simulink model "UAV_Dynamics"  (R2024b)
settings: Solver=ode4  StartTime=0.0  StopTime=10.0  RelTol=1e-3
undefined symbols (not defined in the file): contact, control, ddx, ddy, ddz, dragCoeffMov, dx, dy, dz, fractalcoef, g, m_to_mm, mass, p, pitch, q, r, ref_height, ref_lat, ref_lon, roll, rotorDir, rotorPositions, rotorThrustMax, rotorTimeConst, rotorTorqueMax, SampleTime, windVel, X, Y, yaw, Z
libraries: aerolibatmos2 x1, sensorgpslib x1, robotcorelib x1, mspsensorlib x1, shared6dof x1, simulink x1
settings Model: Creator=The MathWorks, Inc.  LastModifiedBy=davi1
settings SolverCC: ZeroCrossControl=EnableAll  MaxZcPerStep=1
settings OptimizationCC: ReuseModelBlockBuffer=off
settings ModelReferenceCC: EnableRefExpFcnMdlSchedulingChecks=on
settings RTWCC: GPUComputeCapability=3.5  DLArmComputeVersion=19.05

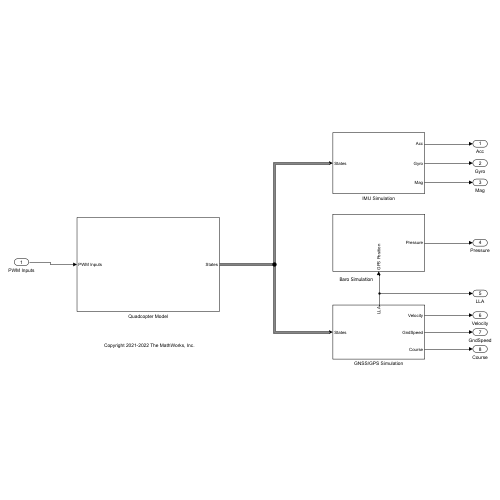
[thumbnail: Simulink's stored preview of the top-level diagram]
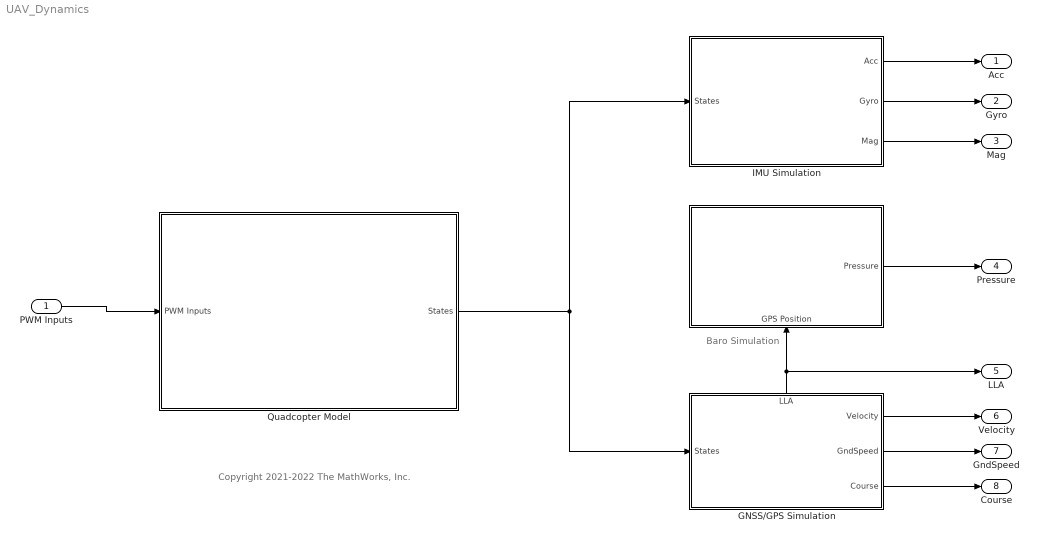
== system UAV_Dynamics ==
  note: Baro Simulation
  note: Copyright 2021-2022 The MathWorks, Inc.
  PWM Inputs : Inport
  " " : Subsystem
      settings: PortSchema="{\"entries\":[{\"content\":{\"sides\":[{\"content\":{\"connectorIds\":[]},\"type\":\"ConnectorPlacement.EquallySpacedRectSide\",\"uuid\":\"7ecc8b21-8f8f-4144-826a-6b68e30dbf7d\"},{\"content\":{\"connectorIds\":[\"Out1\"],\"side\":\"RIGHT\"},\"type\":\"ConnectorPlacement.EquallySpacedRectSide\",\"uuid\":\"81a1dd55-8330-4386-9921-36c0eb60d526\"},{\"content\":{\"connectorIds\":[],\"side\":\"TOP\"},\"type\":\"ConnectorPlacement.EquallySpacedRectSide\",\"uuid\":\"b99caff5-b40d-407d-b30e-35210c1aee1d\"},{\"content\":{\"connectorIds\":[\"In1\"],\"side\":\"BOTTOM\"},\"type\":\"ConnectorPlacement.EquallySpacedRectSide\",\"uuid\":\"18bfda3d-4fab-4e61-9ebc-e384e51de306\"}]},\"type\":\"ConnectorPlacement.EquallySpacedConnector\",\"uuid\":\"17ab4e96-b761-4c62-a0bb-ab626dac3eaa\"}],\"packageUris\":[\"http://schema.mathworks.com/mf0/Connector/R2020b\"],\"version\":\"1.0\"}"
  GNSS/GPS Simulation : Subsystem
      settings: PortSchema="{\"entries\":[{\"content\":{\"sides\":[{\"content\":{\"connectorIds\":[\"In1\"]},\"type\":\"ConnectorPlacement.EquallySpacedRectSide\",\"uuid\":\"4934e8ff-5d4b-4e11-968d-c23bd62383a0\"},{\"content\":{\"connectorIds\":[\"Out1\",\"Out2\",\"Out3\"],\"side\":\"RIGHT\"},\"type\":\"ConnectorPlacement.EquallySpacedRectSide\",\"uuid\":\"9ec8bc0a-2d3c-4dca-835c-010ac29b6ebc\"},{\"content\":{\"connectorIds\":[\"Out4\"],\"side\":\"TOP\"},\"type\":\"ConnectorPlacement.EquallySpacedRectSide\",\"uuid\":\"04f09eb4-1bd9-450e-b951-47054bdd92ad\"}]},\"type\":\"ConnectorPlacement.EquallySpacedConnector\",\"uuid\":\"9a5920cf-a58d-4c98-839b-fbac94edbe7e\"}],\"packageUris\":[\"http://schema.mathworks.com/mf0/Connector/R2020b\"],\"version\":\"1.0\"}"
  IMU Simulation : Subsystem
  Quadcopter Model : Subsystem
  Acc : Outport
  Gyro : Outport  Port=2
  Mag : Outport  Port=3
  Pressure : Outport  Port=4
  LLA : Outport  Port=5
  Velocity : Outport  Port=6
  GndSpeed : Outport  Port=7
  Course : Outport  Port=8
  wires:
  Quadcopter Model/1(States) -> IMU Simulation/1(States), GNSS/GPS Simulation/1(States)
  PWM Inputs/1 -> Quadcopter Model/1(PWM Inputs)
  IMU Simulation/1(Acc) -> Acc/1
  IMU Simulation/2(Gyro) -> Gyro/1
  IMU Simulation/3(Mag) -> Mag/1
  " "/1(Pressure) -> Pressure/1
  GNSS/GPS Simulation/1(Velocity) -> Velocity/1
  GNSS/GPS Simulation/2(GndSpeed) -> GndSpeed/1
  GNSS/GPS Simulation/3(Course) -> Course/1
  GNSS/GPS Simulation/4(LLA) -> LLA/1, " "/1(GPS Position)

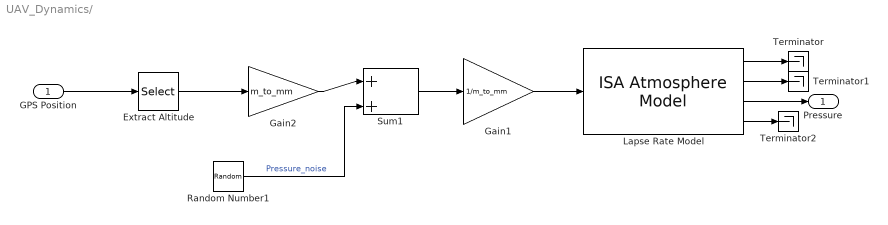
== system UAV_Dynamics/  ==
  GPS Position : Inport
  Extract Altitude : Selector  InputPortWidth=3  IndexOptions=Index vector (dialog)  Indices=[3]  OutputSizes=1
  Gain1 : Gain  Gain=1/m_to_mm
  Gain2 : Gain  Gain=m_to_mm
  Lapse Rate Model : aerolibatmos2/ISA Atmosphere Model  useExtended=off  action=Warning  custom=on  viscosityOut=off  g=9.80665  gamma=1.4  R=287.0531  L=0.0065  h_trop=11000  h_strat=20000  rho0=1.225  P0=101325  T0=288.15  h0=0  S=110.4  Tref=273.15  muref=1.716e-5
  Random Number1 : RandomNumber  Variance=10000  Seed=10  SampleTime=SampleTime
  Sum1 : Sum  Inputs=|++
  Terminator : Terminator
  Terminator1 : Terminator
  Terminator2 : Terminator
  Pressure : Outport
  wires:
  Lapse Rate Model/2 -> Terminator1/1
  Lapse Rate Model/4 -> Terminator2/1
  Lapse Rate Model/1 -> Terminator/1
  Lapse Rate Model/3 -> Pressure/1
  Sum1/1 -> Gain1/1
  Gain2/1 -> Sum1/1
  Extract Altitude/1 -> Gain2/1
  Gain1/1 -> Lapse Rate Model/1
  GPS Position/1 -> Extract Altitude/1
  Random Number1/1 -> Sum1/2  "Pressure_noise"

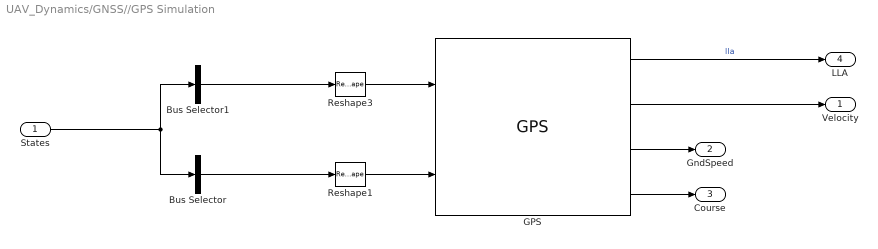
== system UAV_Dynamics/GNSS//GPS Simulation ==
  States : Inport
  Bus Selector : BusSelector  OutputSignals=dx,dy,dz  OutputAsBus=on
  Bus Selector1 : BusSelector  OutputSignals=X,Y,Z  OutputAsBus=on
  GPS : sensorgpslib/GPS  DispRefFrame=NED  PositionInputFormat=Local  ReferenceLocation=[ref_lat ref_lon ref_height]  HorizontalPositionAccuracy=0.01  VerticalPositionAccuracy=0.01  VelocityAccuracy=0.01  DecayFactor=0.99  SeedDouble=67  SimulateUsing=Interpreted execution
  Reshape1 : Reshape  OutputDimensionality=Row vector (2-D)
  Reshape3 : Reshape  OutputDimensionality=Row vector (2-D)
  Velocity : Outport
  GndSpeed : Outport  Port=2
  Course : Outport  Port=3
  LLA : Outport  Port=4
  wires:
  Reshape3/1 -> GPS/1
  GPS/1 -> LLA/1  "lla"
  Bus Selector1/1 -> Reshape3/1
  Bus Selector/1 -> Reshape1/1
  Reshape1/1 -> GPS/2
  GPS/2 -> Velocity/1
  States/1 -> Bus Selector/1, Bus Selector1/1
  GPS/3 -> GndSpeed/1
  GPS/4 -> Course/1

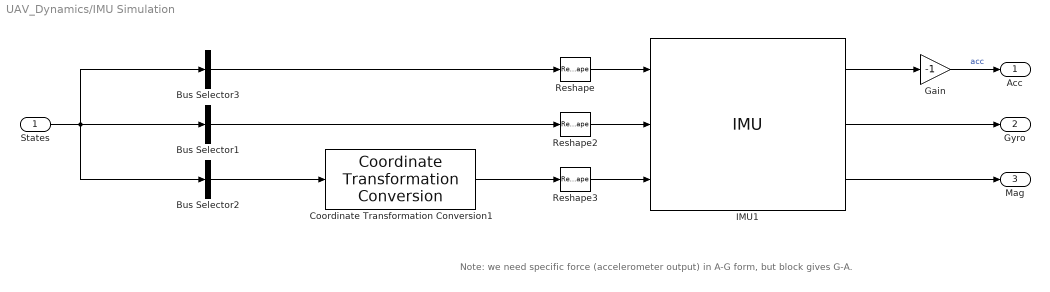
== system UAV_Dynamics/IMU Simulation ==
  note: Note:
      | we need specific force (accelerometer output) in A-G form, but block gives G-A.
  States : Inport
  Bus Selector1 : BusSelector  OutputSignals=p,q,r  OutputAsBus=on
  Bus Selector2 : BusSelector  OutputSignals=yaw,pitch,roll  OutputAsBus=on
  Bus Selector3 : BusSelector  OutputSignals=ddx,ddy,ddz  OutputAsBus=on
  Coordinate Transformation Conversion1 : robotcorelib/Coordinate Transformation Conversion  InputRepresentation=Euler Angles  InputEulerSequence=ZYX  ShowTrVecInputPort=on  OutputRepresentation=Quaternion  OutputEulerSequence=ZYX  ShowTrVecOutputPort=on  SimulateUsing=Interpreted execution
  Gain : Gain  Gain=-1
  IMU1 : mspsensorlib/IMU  DispRefFrame=NED  TemperaturePort=off  Temperature=25  MagneticFieldPort=off  MagneticFieldNED=[21.5 1.16 43.1]  MagneticFieldENU=[ -2.4169, 27.5550, 16.0849 ]  SeedDouble=87254  SimulateUsing=Interpreted execution  AccelParamsMeasurementRange=Inf  AccelParamsResolution=0  AccelParamsConstantBias=[ 0, 0, 0 ]  AccelParamsAxesMisalignment=[ 0, 0, 0 ]  AccelParamsNoiseDensity=0.0003  AccelParamsBiasInstability=[ 0, 0, 0 ]  AccelParamsBiasInstabilityNumerator=fractalcoef().Numerator  AccelParamsBiasInstabilityDenominator=fractalcoef().Denominator  AccelParamsRandomWalk=[ 0, 0, 0 ]  AccelParamsNoiseType=double-sided  AccelParamsTemperatureBias=[ 0, 0, 0 ]  AccelParamsTemperatureScaleFactor=[ 0, 0, 0 ]  GyroParamsMeasurementRange=Inf  GyroParamsResolution=0  GyroParamsConstantBias=[ 0, 0, 0 ]  GyroParamsAxesMisalignment=[ 0, 0, 0 ]  GyroParamsAccelerationBias=0.0001  GyroParamsNoiseDensity=0.01  GyroParamsBiasInstability=[ 0, 0, 0 ]  GyroParamsBiasInstabilityNumerator=fractalcoef().Numerator  GyroParamsBiasInstabilityDenominator=fractalcoef().Denominator  GyroParamsRandomWalk=[ 0, 0, 0 ]  GyroParamsNoiseType=double-sided  GyroParamsTemperatureBias=[ 0, 0, 0 ]  GyroParamsTemperatureScaleFactor=[ 0, 0, 0 ]  MagParamsMeasurementRange=Inf  MagParamsResolution=0  MagParamsConstantBias=[ 0, 0, 0 ]  MagParamsAxesMisalignment=[ 0, 0, 0 ]  MagParamsNoiseDensity=0.0005  MagParamsBiasInstability=[ 0, 0, 0 ]  MagParamsBiasInstabilityNumerator=fractalcoef().Numerator  MagParamsBiasInstabilityDenominator=fractalcoef().Denominator  MagParamsRandomWalk=[ 0, 0, 0 ]  MagParamsNoiseType=double-sided  MagParamsTemperatureBias=[ 0, 0, 0 ]  MagParamsTemperatureScaleFactor=[ 0, 0, 0 ]
  Reshape : Reshape  OutputDimensionality=Row vector (2-D)
  Reshape2 : Reshape  OutputDimensionality=Row vector (2-D)
  Reshape3 : Reshape  OutputDimensionality=Row vector (2-D)
  Acc : Outport
  Gyro : Outport  Port=2
  Mag : Outport  Port=3
  wires:
  Coordinate Transformation Conversion1/1 -> Reshape3/1
  Reshape3/1 -> IMU1/3
  IMU1/3 -> Mag/1
  IMU1/2 -> Gyro/1
  Reshape/1 -> IMU1/1
  Bus Selector3/1 -> Reshape/1
  IMU1/1 -> Gain/1
  Bus Selector1/1 -> Reshape2/1
  Bus Selector2/1 -> Coordinate Transformation Conversion1/1
  Reshape2/1 -> IMU1/2
  States/1 -> Bus Selector1/1, Bus Selector2/1, Bus Selector3/1
  Gain/1 -> Acc/1  "acc"

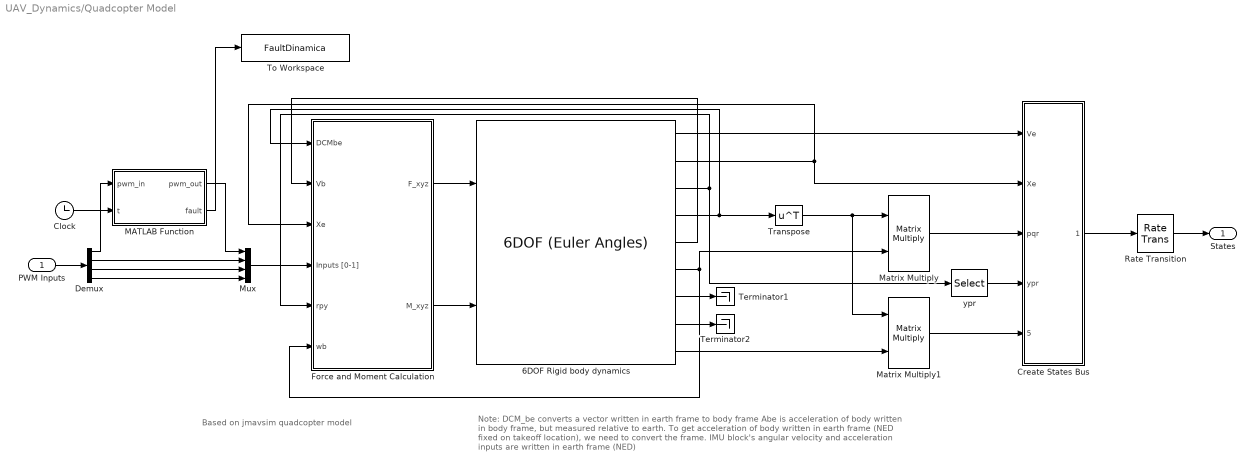
== system UAV_Dynamics/Quadcopter Model ==
  note: Note:
      | DCM_be converts a vector written in earth frame to body frame
      | Abe is acceleration of body written in body frame, but measured relative to earth.
      | To get acceleration of body written in earth frame (NED fixed on takeoff location), we need to convert the frame.
      | IMU block's angular velocity and acceleration inputs are written in earth frame (NED)
  note: Based on jmavsim quadcopter model
  PWM Inputs : Inport
  "6DOF Rigid body dynamics " : shared6dof/6DOF (Euler Angles)  units=Metric (MKS)  mtype=Fixed  rep=Quaternion  xme_0=init.posNED  Vm_0=init.vb  eul_0=init.euler  pm_0=init.angRates  mass_0=mass  mass_e=0.5  mass_f=2.0  inertia=inertia  inertia_e=eye(3)  inertia_f=2*eye(3)  k_quat=1  vre_flag=on  abi_flag=on  aMode=aMode  xme_statename=''  Vm_statename=''  eul_statename=''  quat_statename=''  pm_statename=''  mass_statename=''
  Clock : Clock
  Create States Bus : Subsystem
  Demux : Demux
  Force and Moment Calculation : Subsystem
  MATLAB Function : MATLAB Function  TreatAsAtomicUnit=on
  Matrix Multiply : Product  Multiplication=Matrix(*)
  Matrix Multiply1 : Product  Multiplication=Matrix(*)
  Mux : Mux
  Rate Transition : RateTransition  OutPortSampleTime=SampleTime
  Terminator1 : Terminator
  Terminator2 : Terminator
  To Workspace : ToWorkspace  VariableName=FaultDinamica  SaveFormat=Structure With Time  SampleTime=-1
  Transpose : Math  Operator=transpose
  ypr : Selector  InputPortWidth=3  IndexOptions=Index vector (dialog)  Indices=[3 2 1]  OutputSizes=1
  States : Outport
  wires:
  Matrix Multiply/1 -> Create States Bus/3(pqr)
  "6DOF Rigid body dynamics "/6 -> Matrix Multiply/2, Force and Moment Calculation/6(wb)
  Force and Moment Calculation/1(F_xyz) -> "6DOF Rigid body dynamics "/1
  "6DOF Rigid body dynamics "/9 -> Matrix Multiply1/2
  Transpose/1 -> Matrix Multiply1/1, Matrix Multiply/1
  "6DOF Rigid body dynamics "/5 -> Force and Moment Calculation/2(Vb)
  ypr/1 -> Create States Bus/4(ypr)
  "6DOF Rigid body dynamics "/2 -> Force and Moment Calculation/3(Xe), Create States Bus/2(Xe)
  "6DOF Rigid body dynamics "/3 -> Force and Moment Calculation/5(rpy), ypr/1
  Rate Transition/1 -> States/1
  Create States Bus/1(States) -> Rate Transition/1
  "6DOF Rigid body dynamics "/7 -> Terminator1/1
  "6DOF Rigid body dynamics "/1 -> Create States Bus/1(Ve)
  "6DOF Rigid body dynamics "/8 -> Terminator2/1
  Force and Moment Calculation/2(M_xyz) -> "6DOF Rigid body dynamics "/2
  "6DOF Rigid body dynamics "/4 -> Force and Moment Calculation/1(DCMbe), Transpose/1
  Matrix Multiply1/1 -> Create States Bus/5(acc_lnav)
  PWM Inputs/1 -> Demux/1
  Mux/1 -> Force and Moment Calculation/4(Inputs [0-1])
  Demux/4 -> Mux/4
  Demux/3 -> Mux/3
  Demux/2 -> Mux/2
  MATLAB Function/1(pwm_out) -> Mux/1
  Demux/1 -> MATLAB Function/1(pwm_in)
  Clock/1 -> MATLAB Function/2(t)
  MATLAB Function/2(fault) -> To Workspace/1

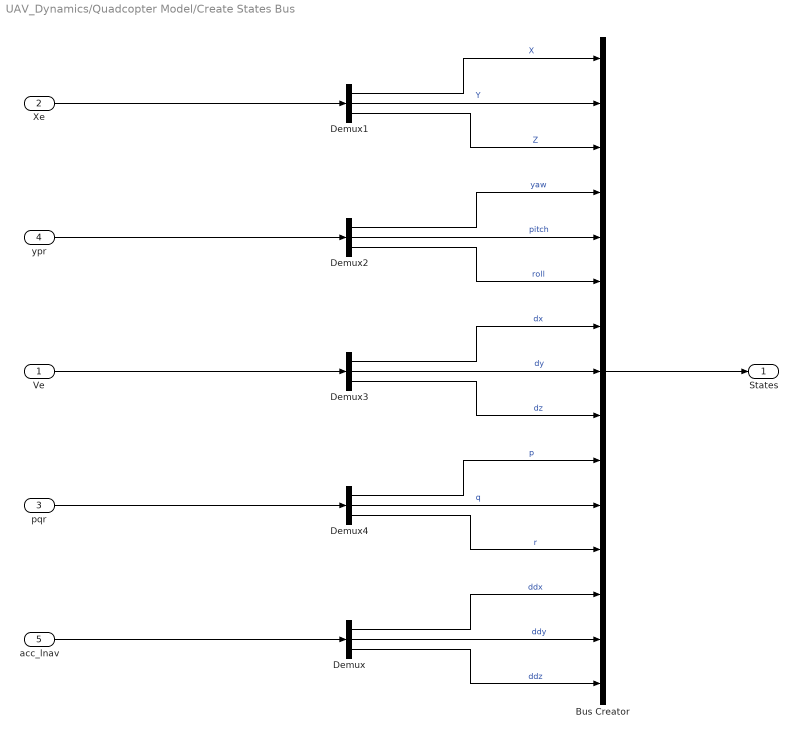
== system UAV_Dynamics/Quadcopter Model/Create States Bus ==
  Ve : Inport
  Xe : Inport  Port=2
  pqr : Inport  Port=3
  ypr : Inport  Port=4
  acc_lnav : Inport  Port=5
  Bus Creator : BusCreator  Inputs=X,Y,Z,yaw,pitch,roll,dx,dy,dz,p,q,r,ddx,ddy,ddz
  Demux{,1..4} (5 alike) : Demux  Outputs=3
  States : Outport
  wires:
  Demux1/1 -> Bus Creator/1  "X"
  Demux1/2 -> Bus Creator/2  "Y"
  ypr/1 -> Demux2/1
  Demux2/2 -> Bus Creator/5  "pitch"
  Demux3/2 -> Bus Creator/8  "dy"
  Demux2/3 -> Bus Creator/6  "roll"
  pqr/1 -> Demux4/1
  Ve/1 -> Demux3/1
  Demux2/1 -> Bus Creator/4  "yaw"
  Demux1/3 -> Bus Creator/3  "Z"
  Demux3/1 -> Bus Creator/7  "dx"
  Demux4/2 -> Bus Creator/11  "q"
  Demux3/3 -> Bus Creator/9  "dz"
  Demux4/3 -> Bus Creator/12  "r"
  Demux4/1 -> Bus Creator/10  "p"
  Bus Creator/1 -> States/1
  Xe/1 -> Demux1/1
  acc_lnav/1 -> Demux/1
  Demux/3 -> Bus Creator/15  "ddz"
  Demux/2 -> Bus Creator/14  "ddy"
  Demux/1 -> Bus Creator/13  "ddx"

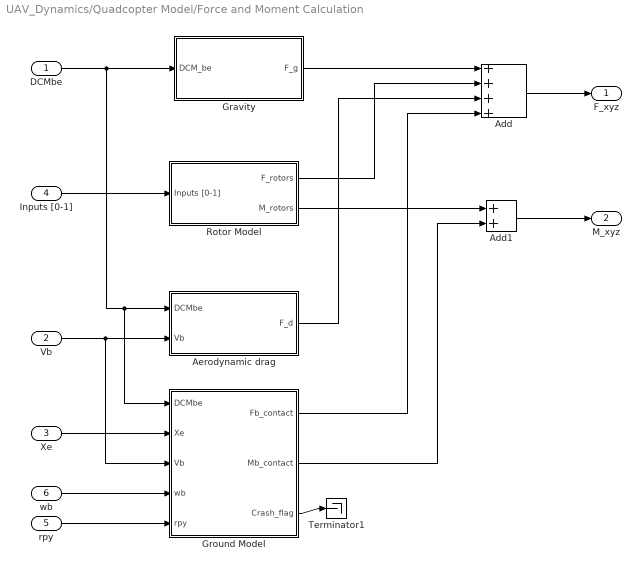
== system UAV_Dynamics/Quadcopter Model/Force and Moment Calculation ==
  DCMbe : Inport
  Vb : Inport  Port=2
  Xe : Inport  Port=3
  Inputs [0-1] : Inport  Port=4
  rpy : Inport  Port=5
  wb : Inport  Port=6
  Add : Sum  Inputs=++++
  Add1 : Sum
  Aerodynamic drag : Subsystem
  Gravity : Subsystem
  Ground Model : Subsystem
  Rotor Model : Subsystem
  Terminator1 : Terminator
  F_xyz : Outport
  M_xyz : Outport  Port=2
  wires:
  Inputs [0-1]/1 -> Rotor Model/1(Inputs [0-1])
  DCMbe/1 -> Ground Model/1(DCMbe), Aerodynamic drag/1(DCMbe), Gravity/1(DCM_be)
  Gravity/1(F_g) -> Add/1
  Add/1 -> F_xyz/1
  Vb/1 -> Ground Model/3(Vb), Aerodynamic drag/2(Vb)
  Rotor Model/1(F_rotors) -> Add/2
  Aerodynamic drag/1(F_d) -> Add/3
  Xe/1 -> Ground Model/2(Xe)
  wb/1 -> Ground Model/4(wb)
  rpy/1 -> Ground Model/5(rpy)
  Rotor Model/2(M_rotors) -> Add1/1
  Ground Model/2(Mb_contact) -> Add1/2
  Add1/1 -> M_xyz/1
  Ground Model/1(Fb_contact) -> Add/4
  Ground Model/3(Crash_flag) -> Terminator1/1

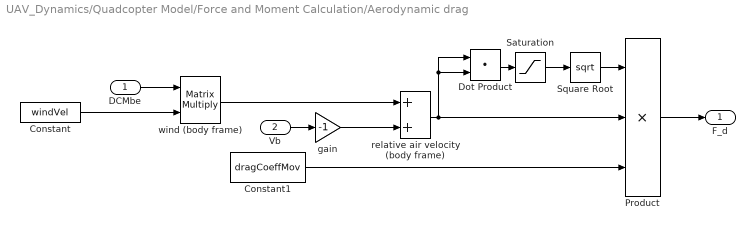
== system UAV_Dynamics/Quadcopter Model/Force and Moment Calculation/Aerodynamic drag ==
  DCMbe : Inport
  Vb : Inport  Port=2
  Constant : Constant  Value=windVel
  Constant1 : Constant  Value=dragCoeffMov
  Dot Product : DotProduct  OutDataTypeStr=Inherit: Inherit via internal rule
  Product : Product  Inputs=3
  Saturation : Saturate  UpperLimit=inf  LowerLimit=0.0001
  Square Root : Sqrt
  gain : Gain  Gain=-1
  relative air velocity (body frame) : Sum
  wind (body frame) : Product  Multiplication=Matrix(*)
  F_d : Outport
  wires:
  relative air velocity (body frame)/1 -> Dot Product/2, Dot Product/1, Product/2
  DCMbe/1 -> wind (body frame)/1
  Product/1 -> F_d/1
  Saturation/1 -> Square Root/1
  Vb/1 -> gain/1
  Dot Product/1 -> Saturation/1
  Square Root/1 -> Product/1
  wind (body frame)/1 -> relative air velocity (body frame)/1
  gain/1 -> relative air velocity (body frame)/2
  Constant1/1 -> Product/3
  Constant/1 -> wind (body frame)/2

== system UAV_Dynamics/Quadcopter Model/Force and Moment Calculation/Gravity ==
  DCM_be : Inport
  Constant : Constant  Value=[0 0 g]'
  Gain : Gain  Gain=mass
  Matrix Multiply : Product  Multiplication=Matrix(*)
  F_g : Outport
  wires:
  Matrix Multiply/1 -> Gain/1
  Constant/1 -> Matrix Multiply/2
  DCM_be/1 -> Matrix Multiply/1
  Gain/1 -> F_g/1

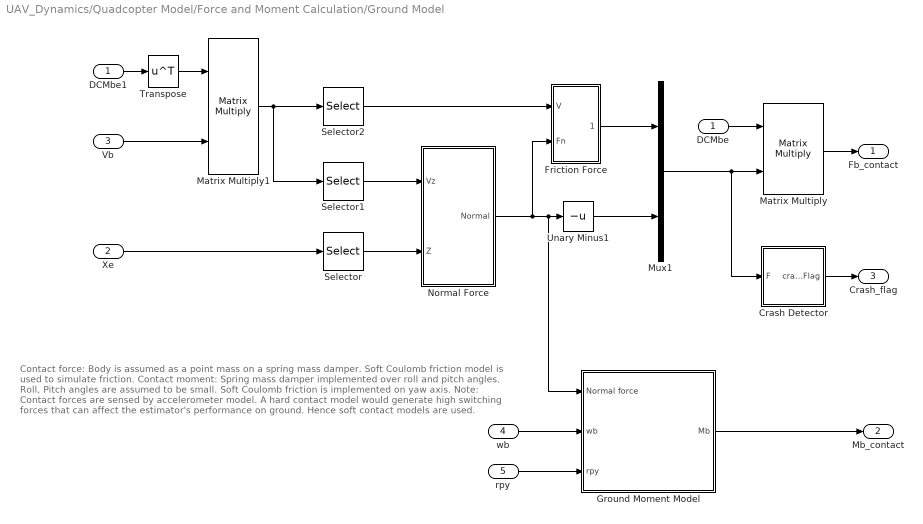
== system UAV_Dynamics/Quadcopter Model/Force and Moment Calculation/Ground Model ==
  note: Contact force:
      | Body is assumed as a point mass on a spring mass damper. Soft Coulomb friction model is used to simulate friction.
      |
      | Contact moment:
      | Spring mass damper implemented over roll and pitch angles. Roll, Pitch angles are assumed to be small.
      | Soft Coulomb friction is implemented on yaw axis.
      |
      | Note:
      | Contact forces are sensed by accelerometer model. A hard contact model would generate high switching forces that can affect the estimator's performance on ground. Hence soft contact models are used.
  DCMbe : Inport
  Xe : Inport  Port=2
  Vb : Inport  Port=3
  wb : Inport  Port=4
  rpy : Inport  Port=5
  Crash Detector : Subsystem
  DCMbe1 : InportShadow
  Friction Force : Subsystem
  Ground Moment Model : Subsystem
  Matrix Multiply : Product  Multiplication=Matrix(*)
  Matrix Multiply1 : Product  Multiplication=Matrix(*)
  Mux1 : Mux  Inputs=2
  Normal Force : Subsystem
  Selector : Selector  InputPortWidth=3  IndexOptions=Index vector (dialog)  Indices=[3]  OutputSizes=1
  Selector1 : Selector  InputPortWidth=3  IndexOptions=Index vector (dialog)  Indices=[3]  OutputSizes=1
  Selector2 : Selector  InputPortWidth=3  IndexOptions=Index vector (dialog)  Indices=[1,2]  OutputSizes=1
  Transpose : Math  Operator=transpose
  Unary Minus1 : UnaryMinus
  Fb_contact : Outport
  Mb_contact : Outport  Port=2
  Crash_flag : Outport  Port=3
  wires:
  Crash Detector/1(crashFlag) -> Crash_flag/1
  Xe/1 -> Selector/1
  Selector1/1 -> Normal Force/1(Vz)
  Selector/1 -> Normal Force/2(Z)
  DCMbe/1 -> Matrix Multiply/1
  Matrix Multiply/1 -> Fb_contact/1
  Normal Force/1(Normal) -> Ground Moment Model/1(Normal force), Unary Minus1/1, Friction Force/2(Fn)
  Mux1/1 -> Crash Detector/1(F), Matrix Multiply/2
  Unary Minus1/1 -> Mux1/2
  Selector2/1 -> Friction Force/1(V)
  Friction Force/1(Friction) -> Mux1/1
  DCMbe1/1 -> Transpose/1
  Transpose/1 -> Matrix Multiply1/1
  Vb/1 -> Matrix Multiply1/2
  Matrix Multiply1/1 -> Selector1/1, Selector2/1
  wb/1 -> Ground Moment Model/2(wb)
  rpy/1 -> Ground Moment Model/3(rpy)
  Ground Moment Model/1(Mb) -> Mb_contact/1

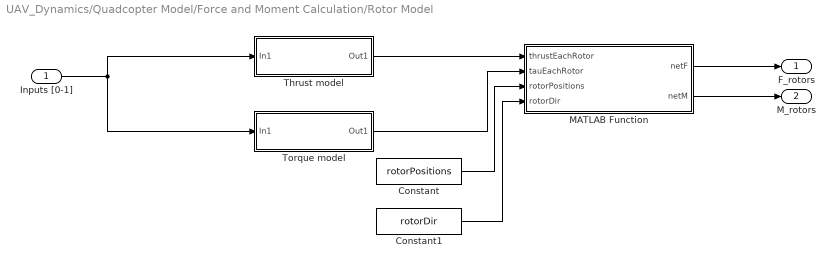
== system UAV_Dynamics/Quadcopter Model/Force and Moment Calculation/Rotor Model ==
  Inputs [0-1] : Inport
  Constant : Constant  Value=rotorPositions
  Constant1 : Constant  Value=rotorDir
  MATLAB Function : MATLAB Function  TreatAsAtomicUnit=on
  Thrust model : Subsystem
  Torque model : Subsystem
  F_rotors : Outport
  M_rotors : Outport  Port=2
  wires:
  Inputs [0-1]/1 -> Torque model/1(In1), Thrust model/1(In1)
  MATLAB Function/1(netF) -> F_rotors/1
  MATLAB Function/2(netM) -> M_rotors/1
  Constant/1 -> MATLAB Function/3(rotorPositions)
  Constant1/1 -> MATLAB Function/4(rotorDir)
  Torque model/1(Out1) -> MATLAB Function/2(tauEachRotor)
  Thrust model/1(Out1) -> MATLAB Function/1(thrustEachRotor)

== system UAV_Dynamics/Quadcopter Model/Force and Moment Calculation/Ground Model/Crash Detector ==
  F : Inport
  Compare To Constant : simulink/Logic and Bit Operations/Compare To Constant  relop=>  const=100  OutDataTypeStr=boolean
  Gain : Gain  Gain=1/mass/g
  norm1 : Subsystem
  crashFlag : Outport
  wires:
  F/1 -> norm1/1(F)
  norm1/1(Out1) -> Gain/1
  Compare To Constant/1 -> crashFlag/1
  Gain/1 -> Compare To Constant/1  "g's"

== system UAV_Dynamics/Quadcopter Model/Force and Moment Calculation/Ground Model/Friction Force ==
  V : Inport
  Fn : Inport  Port=2
  Product : Product
  Saturation : Saturate  UpperLimit=contact.translation.maxFriction  LowerLimit=-contact.translation.maxFriction
  Soft Coulomb Friction : Subsystem
  Unary Minus : UnaryMinus
  Friction : Outport
  wires:
  Fn/1 -> Product/2
  Soft Coulomb Friction/1(Out1) -> Product/1
  Product/1 -> Unary Minus/1
  V/1 -> Soft Coulomb Friction/1(In1)
  Unary Minus/1 -> Saturation/1
  Saturation/1 -> Friction/1

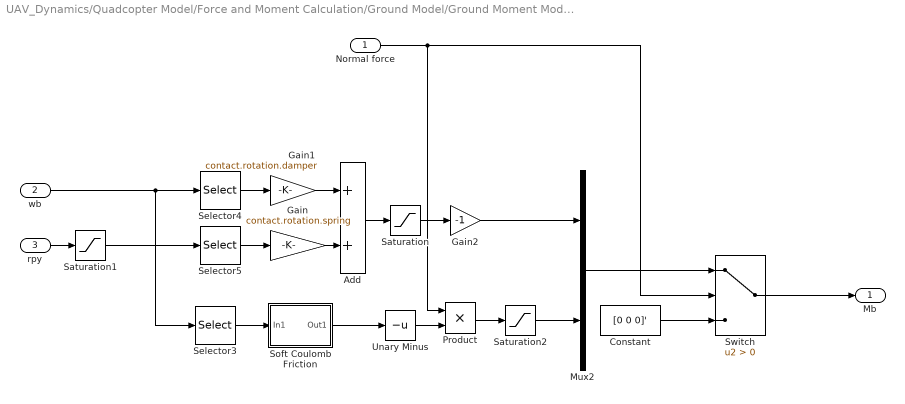
== system UAV_Dynamics/Quadcopter Model/Force and Moment Calculation/Ground Model/Ground Moment Model ==
  Normal force : Inport
  wb : Inport  Port=2
  rpy : Inport  Port=3
  Add : Sum
  Constant : Constant  Value=[0 0 0]'
  Gain : Gain  Gain=contact.rotation.spring
  Gain1 : Gain  Gain=contact.rotation.damper
  Gain2 : Gain  Gain=-1
  Mux2 : Mux  Inputs=2
  Product : Product
  Saturation : Saturate  UpperLimit=control.rotation.maxMoment  LowerLimit=-control.rotation.maxMoment
  Saturation1 : Saturate  UpperLimit=20*pi/180  LowerLimit=-20*pi/180
  Saturation2 : Saturate  UpperLimit=control.rotation.maxMoment  LowerLimit=-control.rotation.maxMoment
  Selector3 : Selector  InputPortWidth=3  IndexOptions=Index vector (dialog)  Indices=[3]  OutputSizes=1
  Selector4 : Selector  InputPortWidth=3  IndexOptions=Index vector (dialog)  Indices=[1, 2]  OutputSizes=1
  Selector5 : Selector  InputPortWidth=3  IndexOptions=Index vector (dialog)  Indices=[1, 2]  OutputSizes=1
  Soft Coulomb Friction : Subsystem
  Switch : Switch  Criteria=u2 > Threshold  SaturateOnIntegerOverflow=off  InputSameDT=off
  Unary Minus : UnaryMinus
  Mb : Outport
  wires:
  Gain2/1 -> Mux2/1
  Add/1 -> Saturation/1
  Gain/1 -> Add/2
  Saturation/1 -> Gain2/1
  Selector4/1 -> Gain1/1
  Gain1/1 -> Add/1
  Constant/1 -> Switch/3
  Selector5/1 -> Gain/1
  Switch/1 -> Mb/1
  Mux2/1 -> Switch/1
  Normal force/1 -> Product/1, Switch/2
  rpy/1 -> Saturation1/1
  Saturation1/1 -> Selector5/1
  wb/1 -> Selector4/1, Selector3/1
  Selector3/1 -> Soft Coulomb Friction/1(In1)
  Soft Coulomb Friction/1(Out1) -> Unary Minus/1
  Unary Minus/1 -> Product/2
  Product/1 -> Saturation2/1
  Saturation2/1 -> Mux2/2

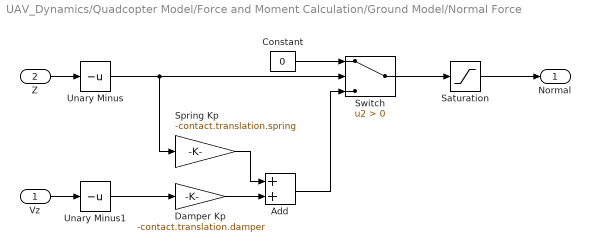
== system UAV_Dynamics/Quadcopter Model/Force and Moment Calculation/Ground Model/Normal Force ==
  Vz : Inport
  Z : Inport  Port=2
  Add : Sum
  Constant : Constant  Value=0
  Damper Kp : Gain  Gain=-contact.translation.damper
  Saturation : Saturate  UpperLimit=contact.translation.maxNormal  LowerLimit=0
  Spring Kp : Gain  Gain=-contact.translation.spring
  Switch : Switch  Criteria=u2 > Threshold  SaturateOnIntegerOverflow=off  InputSameDT=off
  Unary Minus : UnaryMinus
  Unary Minus1 : UnaryMinus
  Normal : Outport
  wires:
  Constant/1 -> Switch/1
  Z/1 -> Unary Minus/1
  Switch/1 -> Saturation/1
  Damper Kp/1 -> Add/2
  Add/1 -> Switch/3
  Spring Kp/1 -> Add/1
  Vz/1 -> Unary Minus1/1
  Saturation/1 -> Normal/1
  Unary Minus/1 -> Spring Kp/1, Switch/2
  Unary Minus1/1 -> Damper Kp/1

== system UAV_Dynamics/Quadcopter Model/Force and Moment Calculation/Rotor Model/Thrust model ==
  In1 : Inport
  Demux : Demux
  Mux : Mux
  Transfer Fcn{,2..4} (4 alike) : TransferFcn  Numerator=[rotorThrustMax]  Denominator=[rotorTimeConst 1]
  Out1 : Outport
  wires:
  Transfer Fcn3/1 -> Mux/2
  Demux/1 -> Transfer Fcn4/1
  Transfer Fcn2/1 -> Mux/3
  Demux/3 -> Transfer Fcn2/1
  Mux/1 -> Out1/1
  Transfer Fcn4/1 -> Mux/1
  Demux/4 -> Transfer Fcn/1
  Demux/2 -> Transfer Fcn3/1
  Transfer Fcn/1 -> Mux/4
  In1/1 -> Demux/1

== system UAV_Dynamics/Quadcopter Model/Force and Moment Calculation/Rotor Model/Torque model ==
  In1 : Inport
  Demux : Demux
  Mux : Mux
  Transfer Fcn{1..4} (4 alike) : TransferFcn  Numerator=[rotorTorqueMax]  Denominator=[rotorTimeConst 1]
  Out1 : Outport
  wires:
  Transfer Fcn4/1 -> Mux/4
  Demux/1 -> Transfer Fcn1/1
  Transfer Fcn3/1 -> Mux/3
  Transfer Fcn2/1 -> Mux/2
  Demux/2 -> Transfer Fcn2/1
  Demux/4 -> Transfer Fcn4/1
  Demux/3 -> Transfer Fcn3/1
  Mux/1 -> Out1/1
  Transfer Fcn1/1 -> Mux/1
  In1/1 -> Demux/1

== system UAV_Dynamics/Quadcopter Model/Force and Moment Calculation/Ground Model/Crash Detector/norm1 ==
  F : Inport
  Dot Product : DotProduct  OutDataTypeStr=Inherit: Inherit via internal rule
  Sqrt : Sqrt
  Out1 : Outport
  wires:
  Dot Product/1 -> Sqrt/1
  F/1 -> Dot Product/2, Dot Product/1
  Sqrt/1 -> Out1/1

== system UAV_Dynamics/Quadcopter Model/Force and Moment Calculation/Ground Model/Friction Force/Soft Coulomb Friction ==
  note: Pennestrì, E., Rossi, V., Salvini, P. et al. Review and comparison of dry friction force models. Nonlinear Dyn 83, 1785–1801 (2016). https://doi.org/10.1007/s11071-015-2485-3
  In1 : Inport
  Tanh : Trigonometry  Operator=tanh
  friction coefficient : Gain  Gain=contact.translation.friction
  vd : Gain  Gain=1/contact.translation.vd
  Out1 : Outport
  wires:
  In1/1 -> vd/1
  vd/1 -> Tanh/1
  Tanh/1 -> friction coefficient/1
  friction coefficient/1 -> Out1/1

== system UAV_Dynamics/Quadcopter Model/Force and Moment Calculation/Ground Model/Ground Moment Model/Soft Coulomb Friction ==
  note: Pennestrì, E., Rossi, V., Salvini, P. et al. Review and comparison of dry friction force models. Nonlinear Dyn 83, 1785–1801 (2016). https://doi.org/10.1007/s11071-015-2485-3
  In1 : Inport
  Tanh : Trigonometry  Operator=tanh
  friction coefficient : Gain  Gain=control.rotation.friction
  vd : Gain  Gain=1/control.rotation.vd
  Out1 : Outport
  wires:
  In1/1 -> vd/1
  vd/1 -> Tanh/1
  Tanh/1 -> friction coefficient/1
  friction coefficient/1 -> Out1/1

== matlab function UAV_Dynamics/Quadcopter Model/MATLAB Function ==
  data: pwm_in input; pwm_out output; t input; fault output
function [pwm_out, fault] = FaultGain(pwm_in, t) %#codegen
% pwm_in: segnale PWM in ingresso
% t: tempo della simulazione (dal blocco Clock)
double gain;
uint16 fault;

fault = 0;
    if t <= 100
        gain = 1.0;
    elseif t <= 160
        gain = 0.95;
        fault = 1;
    elseif t <= 220
        gain = 0.90;
        fault = 2;
    else
        gain = 0.85;
        fault = 3;
    end
    pwm_out = pwm_in*gain;
end

== matlab function UAV_Dynamics/Quadcopter Model/Force and Moment Calculation/Rotor Model/MATLAB Function ==
  data: thrustEachRotor input; tauEachRotor input; rotorPositions input; netF output; netM output; rotorDir input
function [netF, netM] = getForceMoment(thrustEachRotor, tauEachRotor, rotorPositions, rotorDir)
%#codegen
Fx = 0;
Fy = 0;
Fz = -sum(thrustEachRotor);

netF = [Fx; Fy; Fz];

netM = [0; 0; 0]; %initialize
    for i = 1:4
        rotPos = rotorPositions(:, i);
        Fi = [0, 0, -thrustEachRotor(i)]';
        netM = netM +  cross(rotPos, Fi);%contribution from thrusts of each propeller
        netM(3) = netM(3) - rotorDir(i)*tauEachRotor(i); %contribution from counter torque acting on propeller
    end

end
